simulink model "projemodel1"  (R2019a)
settings: Solver=VariableStepAuto  StartTime=0.0  StopTime=10.0  RelTol=1e-3
settings Model: Creator=tr531  LastModifiedBy=tr531

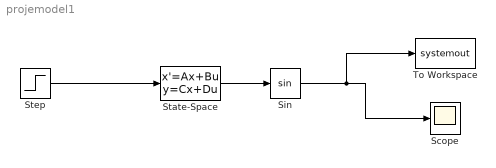
== system projemodel1 ==
  Scope : Scope
  Sin : Trigonometry
  State-Space : StateSpace  A=[1 1 1/2;0 1 1;0 0 1]  B=[0 ; 0; 1/80]  C=[1 0 0]  D=0  InitialCondition=0
  Step : Step  Time=0  After=0.0001  SampleTime=0
  To Workspace : ToWorkspace  VariableName=systemout  SaveFormat=Timeseries  SampleTime=-1
  wires:
  Step/1 -> State-Space/1
  State-Space/1 -> Sin/1
  Sin/1 -> Scope/1, To Workspace/1
